simulink model "Step_12"  (Simulink 7.9)
settings: Solver=ode23  StartTime=0.0  StopTime=500  MaxStep=1  RelTol=1e-3
PostLoadFcn:
  | m = 150;
  | load mybus
libraries: aerolibconvert2 x2, aerolibfltsims x1, simulink x1, drag_library_masked x1, aerolibanimutils x1
settings Model: Creator=wcampbel  LastModifiedBy=wcampbel
settings DebuggingCC: FcnCallInpInsideContextMsg=Use local settings  StrictBusMsg=Warning
settings GRTTargetCC: CombineOutputUpdateFcns=off  GRTInterface=on

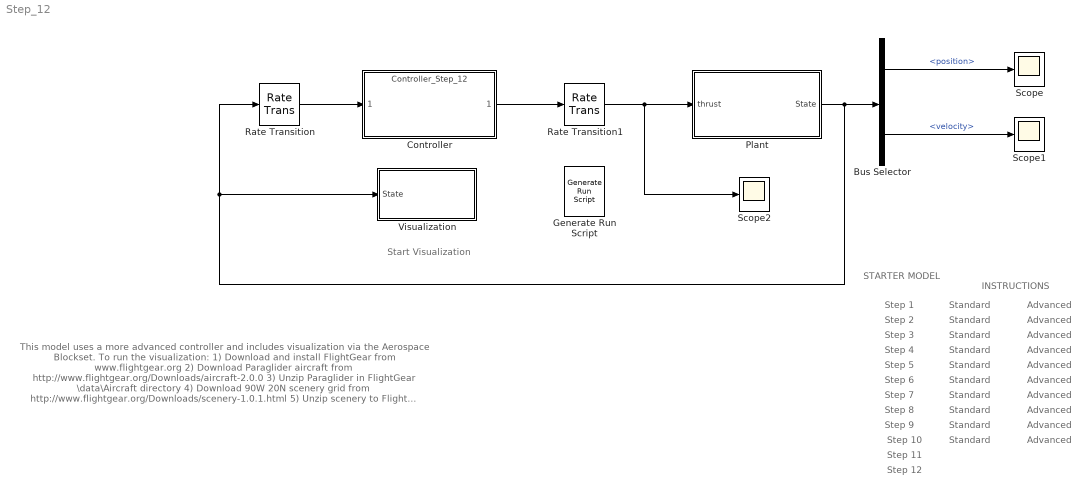
== system Step_12 ==
  note: Step 1
  note: Step 2
  note: Step 3
  note: STARTER
      | MODEL
  note: INSTRUCTIONS
  note: Step 4
  note: Step 5
  note: Step 6
  note: Standard
  note: Advanced
  note: Standard
  note: Advanced
  note: Standard
  note: Advanced
  note: Standard
  note: Standard
  note: Advanced
  note: Standard
  note: Advanced
  note: Step 7
  note: Step 8
  note: Step 9
  note: Step 10
  note: Step 11
  note: Standard
  note: Advanced
  note: Advanced
  note: Advanced
  note: Advanced
  note: Standard
  note: Standard
  note: Standard
  note: Advanced
  note: Start Visualization
  note: This model uses a more advanced controller and includes visualization via the Aerospace Blockset.
      |
      | To run the visualization:
      | 1) Download and install FlightGear from www.flightgear.org
      | 2) Download Paraglider aircraft from http://www.flightgear.org/Downloads/aircraft-2.0.0
      | 3) Unzip Paraglider in FlightGear \data\Aircraft directory
      | 4) Download 90W 20N scenery grid from http://www.flightgear.org/Downloads/scenery-1.0.1.html
      | 5) Unzip scenery to Flight \data\Scenery directory
      | 6) Double-click Generate Run Script, verify that settings are correct, rebuild as necessary
      | 7) Run the visualization script by typing in the MATLAB command window or using model hyperlink
  note: Step 12
  Bus Selector : BusSelector  OutputSignals=position,velocity
  Controller : ModelReference  ModelNameDialog=Controller_Step_12  SimulationMode=Normal  ModelReferenceVersion=1.3  CopyOfModelName=Controller_Step_12  DefaultDataLogging=off
  Generate Run Script : aerolibfltsims/Generate Run Script  OutputFileName=runfg.bat  FlightGearBaseDirectory=C:\Program Files\FlightGear  GeometryModelName=paraglider  DestinationPort=5502  OriginAddress=127.0.0.1  OriginPort=5505  AirportId=KXMR  RunwayId=13  InitialAltitude=3297  InitialHeading=100  OffsetDistance=3.5  OffsetAzimuth=0  GenerateFile=off  Architecture=Default  dataFlow=Send
  Plant : Subsystem
  Rate Transition : RateTransition
  Rate Transition1 : RateTransition
  Scope : Scope
      settings: ShowLegends=on  TimeRange=100  YMin=-1.25  YMax=2.5
  Scope1 : Scope
      settings: ShowLegends=on  TimeRange=100  YMin=0  YMax=250
  Scope2 : Scope
      settings: ShowLegends=on  TimeRange=39.54372623574145  YMin=-98.18359374999955  YMax=1990.625  SaveName=ScopeData2
  Visualization : Subsystem
  wires:
  Plant/1(State) -> Bus Selector/1, Rate Transition/1, Visualization/1(State)
  Controller/1 -> Rate Transition1/1
  Rate Transition/1 -> Controller/1
  Rate Transition1/1 -> Scope2/1, Plant/1(thrust)
  Bus Selector/1 -> Scope/1  "<position>"
  Bus Selector/2 -> Scope1/1  "<velocity>"

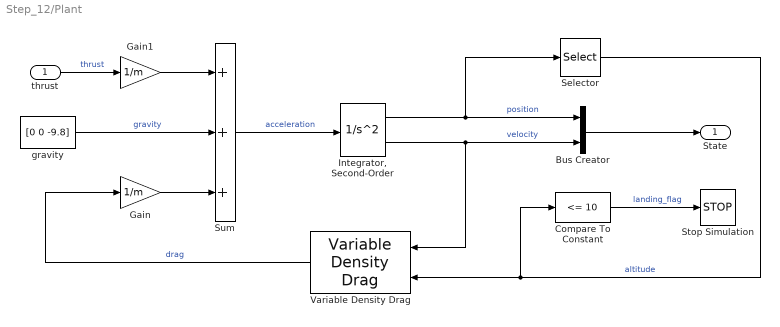
== system Step_12/Plant ==
  thrust : Inport
  Bus Creator : BusCreator  Inputs=2
  Compare To Constant : simulink/Logic and Bit Operations/Compare To Constant  relop=<=  const=10  OutDataTypeStr=boolean
  Gain : Gain  Gain=1/m
  Gain1 : Gain  Gain=1/m
  "Integrator, Second-Order" : SecondOrderIntegrator  ICX=[0 0 1015]  ICDXDT=[1 3 1]
  Selector : Selector  InputPortWidth=3  IndexOptions=Index vector (dialog)  Indices=3  OutputSizes=1
  Stop Simulation : Stop
  Sum : Sum  Inputs=+++
  Variable Density Drag : drag_library_masked/Variable Density Drag  Cd=0.333  A=1.5
  gravity : Constant  Value=[0 0 -9.8]
  State : Outport
  wires:
  "Integrator, Second-Order"/2 -> Variable Density Drag/1, Bus Creator/2  "velocity"
  Variable Density Drag/1 -> Gain/1  "drag"
  Sum/1 -> "Integrator, Second-Order"/1  "acceleration"
  thrust/1 -> Gain1/1  "thrust"
  Gain1/1 -> Sum/1
  gravity/1 -> Sum/2  "gravity"
  Gain/1 -> Sum/3
  Bus Creator/1 -> State/1
  "Integrator, Second-Order"/1 -> Bus Creator/1, Selector/1  "position"
  Selector/1 -> Variable Density Drag/2, Compare To Constant/1  "altitude"
  Compare To Constant/1 -> Stop Simulation/1  "landing_flag"

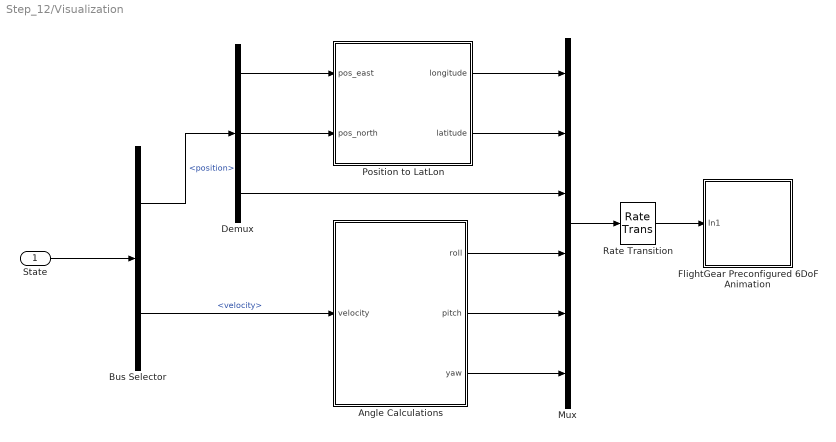
== system Step_12/Visualization ==
  State : Inport
  Angle Calculations : Subsystem
  Bus Selector : BusSelector  OutputSignals=position,velocity
  Demux : Demux  Outputs=3
  FlightGear Preconfigured 6DoF Animation : Subsystem  TreatAsAtomicUnit=on  SimViewingDevice=on  mask(FlightGearQuick6DoFAnimation){xFlightGearVersion=v2.0, DestinationIpAddress=127.0.0.1, DestinationPort=5502, SampleTime=1/30}
      mask prompts: xFlightGearVersion "FlightGear version:"; DestinationIpAddress "Destination IP address:"; DestinationPort "Destination port:"; SampleTime "Sample time (-1 for inherited):"
      mask help:
      | Drive position and attitude values to a FlightGear Flight Simulator vehicle given double precision values for longitude, latitude, altitude, roll, pitch, and yaw respectively.  Units are degrees west/north for longitude and latitude, meters above mean sea level for altitude, and radians for attitude values.
      |
      | This block is a masked subsystem containing principally a FlightGear Pack Net FDM block set for 6DoF inputs, a FlightGear Send Net FDM block, and a Simulation Pace block.  To access the full capabilities of these blocks, use the individual corresponding blocks from the Aerospace Blockset library.
      |
      | Use "Look under mask" from this block's context menu to see the blocks under the mask.
      mask init:
      | [xp, yp] = aeroimage('anim',gcbh);
      | xp = xp * 0.7 + 0.45;
      | yp = yp * 0.7 + 0.45;
      settings: AttributesFormatString=Version Selected: %<xFlightGearVersion>
      mask Help: eval('asbhelp(''flightgear_preconfigured_6dof_animation'')');
      mask StyleString: popup(v0.9.3|v0.9.8|v0.9.9|v0.9.10|v1.0|v1.9.1|v2.0),edit,edit,edit
      mask Display:
      | port_label('input',1,'l,\mu,h,\phi,\theta,\psi','texmode','on')
      | patch(xp,yp)
  Mux : Mux  Inputs=6
  Position to LatLon : Subsystem  mask(Position to Latitude and Longitude Conversion){lat0=28.506, lon0=-80.64105}
      mask prompts: lat0 "Initial Latitude [deg]"; lon0 "Initial Longitude [deg]"
      mask help:
      | This subsystem provides the latitude and longitude of a position on or above the Earth's surface. The user supplies an initial set of coordinates in degrees via the mask. Inputs to the system are the deviation east and north of the coordinate specified in meters.
      |
      | Note that if in the western hemisphere, longitude should be negative.
      mask init:
      | % Define conversion from meters to minutes of longitude based on initial
      | % latitude. Note that the latitude range is limited.
      | 
      | latitude_data     = [30:5:50];
      | meters_per_minute = [1608 1522 1423 1314 1195];
      | 
      | % Find conversion
      | meters_per_lon = interp1(latitude_data,meters_per_minute,lat0,'linear','extrap')*60;
      | 
      | % Define meters per latitude 
      | meters_per_lat = 111118;
  Rate Transition : RateTransition  OutPortSampleTime=1/30
  wires:
  Position to LatLon/2(latitude) -> Mux/2
  Demux/2 -> Position to LatLon/2(pos_north)
  Demux/1 -> Position to LatLon/1(pos_east)
  Position to LatLon/1(longitude) -> Mux/1
  Mux/1 -> Rate Transition/1
  Angle Calculations/1(roll) -> Mux/4
  Angle Calculations/3(yaw) -> Mux/6
  Angle Calculations/2(pitch) -> Mux/5
  Demux/3 -> Mux/3
  Bus Selector/1 -> Demux/1  "<position>"
  Bus Selector/2 -> Angle Calculations/1(velocity)  "<velocity>"
  State/1 -> Bus Selector/1
  Rate Transition/1 -> FlightGear Preconfigured 6DoF Animation/1(In1)

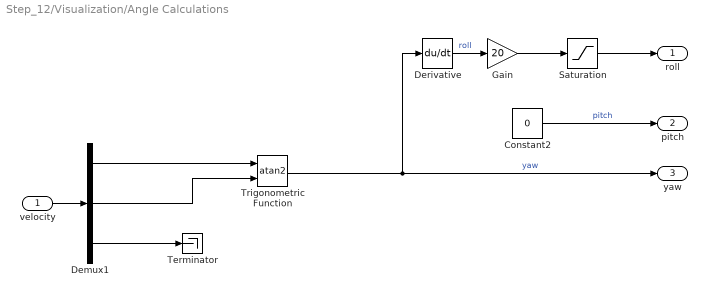
== system Step_12/Visualization/Angle Calculations ==
  velocity : Inport
  Constant2 : Constant  Value=0  SampleTime=0
  Demux1 : Demux  Outputs=3
  Derivative : Derivative
  Gain : Gain  Gain=20
  Saturation : Saturate  UpperLimit=15/180*pi  LowerLimit=-15/180*pi
  Terminator : Terminator
  Trigonometric Function : Trigonometry  Operator=atan2
  roll : Outport
  pitch : Outport  Port=2
  yaw : Outport  Port=3
  wires:
  Demux1/1 -> Trigonometric Function/1
  Demux1/2 -> Trigonometric Function/2
  velocity/1 -> Demux1/1
  Constant2/1 -> pitch/1  "pitch"
  Demux1/3 -> Terminator/1
  Trigonometric Function/1 -> yaw/1, Derivative/1  "yaw"
  Derivative/1 -> Gain/1  "roll"
  Gain/1 -> Saturation/1
  Saturation/1 -> roll/1

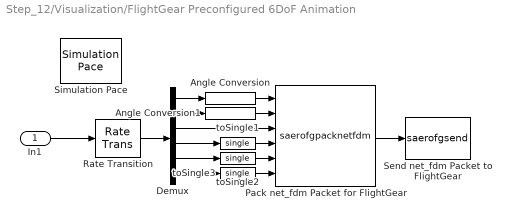
== system Step_12/Visualization/FlightGear Preconfigured 6DoF Animation ==
  In1 : Inport
  Angle Conversion : aerolibconvert2/Angle Conversion  IU=deg  OU=rad
  Angle Conversion1 : aerolibconvert2/Angle Conversion  IU=deg  OU=rad
  Demux : Demux  Outputs=6
  Pack net_fdm Packet for FlightGear : S-Function  FunctionName=saerofgpacknetfdm  Parameters=xFlightGearVersion, 'on','off','off','off','off','off', SampleTime  EnableBusSupport=off
  Rate Transition : RateTransition  Integrity=off  Deterministic=off  OutPortSampleTime=SampleTime
  Send net_fdm Packet to FlightGear : S-Function  InitFcn=|  FunctionName=saerofgsend  Parameters=DestinationIpAddress, DestinationPort, -1, SampleTime,0  EnableBusSupport=off
      | xpctab = {'xpctarget.tlc' 'xpctargetert.tlc'};                                                      
      | sfuntab = {'saerofgsend' 'xpcudpbytesend' 'xpcudpbytesend'};                                        
      | idx = find(strcmp(xpctab,get_param(bdroot,'SystemTargetFile')));                                    
      | if isempty(idx)                                                                                     
      |     if (license('test','xpc_target')&&strcmp(computer,'PCWIN'))                                     
      |         idx = 0;                                                                                    
      |     else                                                                                            
      |         idx = 1;                                                                                    
      |     end                                                                                             
      | end                                                                                                 
      | set_param(gcb,'FunctionName',sfuntab{idx+(license('test','xpc_target')&&strcmp(computer,'PCWIN'))});
  Simulation Pace : aerolibanimutils/Simulation Pace  SimulationPace=3  SleepMode=MATLAB Thread  OutputPaceError=off  SampleTime=SampleTime
      settings: AttributesFormatString=%<SimulationPace> sec/sec
  toSingle1 : DataTypeConversion  OutDataTypeStr=single
  toSingle2 : DataTypeConversion  OutDataTypeStr=single
  toSingle3 : DataTypeConversion  OutDataTypeStr=single
  wires:
  Demux/6 -> toSingle3/1
  Demux/5 -> toSingle2/1
  Demux/4 -> toSingle1/1
  Demux/3 -> Pack net_fdm Packet for FlightGear/3
  Demux/2 -> Angle Conversion1/1
  Demux/1 -> Angle Conversion/1
  In1/1 -> Rate Transition/1
  Pack net_fdm Packet for FlightGear/1 -> Send net_fdm Packet to FlightGear/1
  toSingle1/1 -> Pack net_fdm Packet for FlightGear/4
  toSingle2/1 -> Pack net_fdm Packet for FlightGear/5
  toSingle3/1 -> Pack net_fdm Packet for FlightGear/6
  Rate Transition/1 -> Demux/1
  Angle Conversion/1 -> Pack net_fdm Packet for FlightGear/1
  Angle Conversion1/1 -> Pack net_fdm Packet for FlightGear/2

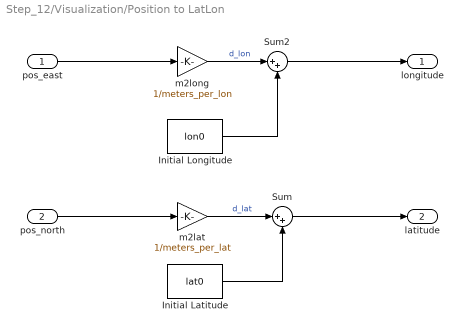
== system Step_12/Visualization/Position to LatLon ==
  pos_east : Inport
  pos_north : Inport  Port=2
  Initial Latitude : Constant  Value=lat0
  Initial Longitude : Constant  Value=lon0
  Sum : Sum  Inputs=|++
  Sum2 : Sum  Inputs=|++
  m2lat : Gain  Gain=1/meters_per_lat
  m2long : Gain  Gain=1/meters_per_lon
  longitude : Outport
  latitude : Outport  Port=2
  wires:
  m2lat/1 -> Sum/1  "d_lat"
  Initial Latitude/1 -> Sum/2
  m2long/1 -> Sum2/1  "d_lon"
  Initial Longitude/1 -> Sum2/2
  pos_north/1 -> m2lat/1
  pos_east/1 -> m2long/1
  Sum2/1 -> longitude/1
  Sum/1 -> latitude/1
